simulink model "ctrlauto_tp1_sim_f"  (R2019b)
settings: Solver=VariableStepAuto  StartTime=0.0  StopTime=5  RelTol=1e-3
undefined symbols (not defined in the file or in its folder): k, ueq, xeq
settings Model: Creator=rochi  LastModifiedBy=rochi

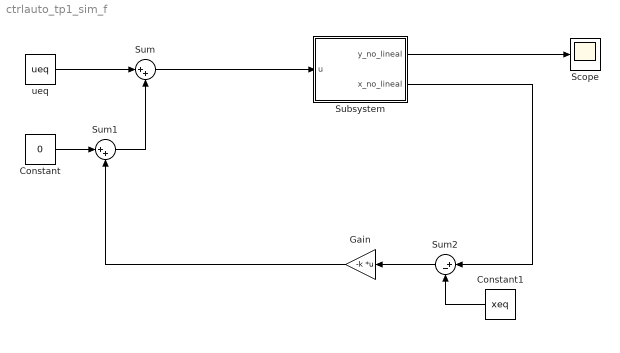
== system ctrlauto_tp1_sim_f ==
  Constant : Constant  Value=0
  Constant1 : Constant  Value=xeq
  Gain : Gain  Gain=-k  Multiplication=Matrix(K*u)
  Scope : Scope
  Subsystem : Subsystem
  Sum : Sum  Inputs=|++
  Sum1 : Sum  Inputs=|++
  Sum2 : Sum  Inputs=|+-
  ueq : Constant  Value=ueq
  wires:
  ueq/1 -> Sum/1
  Sum/1 -> Subsystem/1(u)
  Sum1/1 -> Sum/2
  Constant/1 -> Sum1/1
  Gain/1 -> Sum1/2
  Constant1/1 -> Sum2/2
  Sum2/1 -> Gain/1
  Subsystem/2(x_no_lineal) -> Sum2/1
  Subsystem/1(y_no_lineal) -> Scope/1

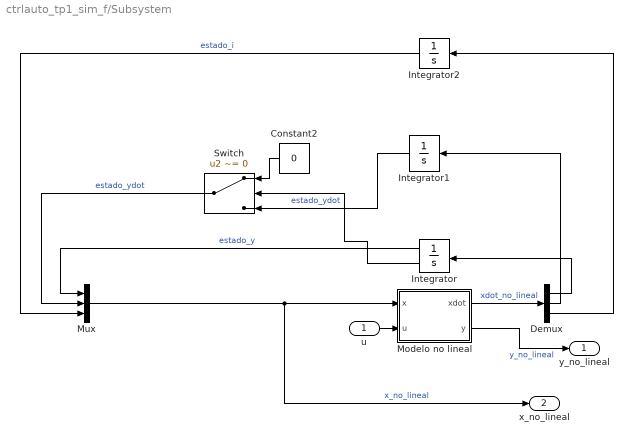
== system ctrlauto_tp1_sim_f/Subsystem ==
  u : Inport
  Constant2 : Constant  Value=0
  Demux : Demux  Outputs=3
  Integrator : Integrator  InitialCondition=0.3  LimitOutput=on  UpperSaturationLimit=.95  LowerSaturationLimit=-0.95  ShowSaturationPort=on
  Integrator1 : Integrator  InitialCondition=0.2  LimitOutput=on  UpperSaturationLimit=1e5  LowerSaturationLimit=-1e5
  Integrator2 : Integrator  InitialCondition=xeq(3)  LimitOutput=on  UpperSaturationLimit=50  LowerSaturationLimit=-50
  Modelo no lineal : MATLAB Function  TreatAsAtomicUnit=on
  Mux : Mux  Inputs=3
  Switch : Switch  Criteria=u2 ~= 0
  y_no_lineal : Outport
  x_no_lineal : Outport  Port=2
  wires:
  Integrator/1 -> Mux/1  "estado_y"
  Demux/3 -> Integrator2/1
  Demux/1 -> Integrator/1
  Integrator/2 -> Switch/2
  Integrator1/1 -> Switch/3  "estado_ydot"
  Mux/1 -> x_no_lineal/1, Modelo no lineal/1(x)  "x_no_lineal"
  Modelo no lineal/1(xdot) -> Demux/1  "xdot_no_lineal"
  Demux/2 -> Integrator1/1
  Switch/1 -> Mux/2  "estado_ydot"
  u/1 -> Modelo no lineal/2(u)
  Integrator2/1 -> Mux/3  "estado_i"
  Constant2/1 -> Switch/1
  Modelo no lineal/2(y) -> y_no_lineal/1  "y_no_lineal"

== matlab function ctrlauto_tp1_sim_f/Subsystem/Modelo no lineal ==
  data: x input; xdot output; u input; y output
function [xdot,y] = nolineal(x, u)
    xdot1 = x(2);
    xdot2 = (5*(x(3) + 2)^2)/(2*(x(1) - 1)^2) - (5*(x(3)  - 2)^2)/(2*(x(1) + 1)^2) - 10; 
    xdot3 = - 4*x(3)^2 + u;

    xdot = [xdot1; xdot2; xdot3];
    y = x(1);
end
